simulink model "mdaqdemo_uart"  (R2014a)
settings: Solver=FixedStepDiscrete  SolverMode=SingleTasking  StartTime=0.0  StopTime=100  FixedStep=0.1  RelTol=1e-3
libraries: microdaq_lib x4, etargetslib x2, simulink x2
settings Model: SimulationMode=external  Creator=skibool  LastModifiedBy=skibool
settings OptimizationCC: OptimizeModelRefInitCode=on  LifeSpan=1
settings DebuggingCC: MergeDetectMultiDrivingBlocksExec=error  FrameProcessingCompatibilityMsg=error
settings HardwareCC: ProdBitPerLong=40  ProdLargestAtomicInteger=Integer  ProdIntDivRoundTo=Zero  ProdEndianess=LittleEndian  ProdHWDeviceType=Texas Instruments->C6000
settings RTWCC: SystemTargetFile=microdaq.tlc  TemplateMakefile=microdaq.tmf  PostCodeGenCommand=microdaq_postcodegen(buildInfo)  Description=MicroDAQ Real-Time Measurement System
settings CodeAppCC: IgnoreCustomStorageClasses=off
settings STFCustomTargetCC: ConcurrentExecutionCompliant=off  GeneratePreprocessorConditionals=Use local settings  CombineOutputUpdateFcns=on  ERTCustomFileBanners=on  SupportContinuousTime=off  SupportNonInlinedSFcns=off  MATLABClassNameForMDSCustomization=Simulink.SoftwareTarget.ERTCustomization  GRTInterface=off  SystemTargetFile=microdaq.tlc
settings ERTTargetCC: GenerateSampleERTMain=off  ExtMode=on  ExtModeStaticAlloc=on  ExtModeStaticAllocSize=1485760  ExtModeMexArgs=getpref('microdaq','TargetIP') 1 4344  InlinedParameterPlacement=Hierarchical  ERTCustomFileTemplate=microdaq_main.tlc

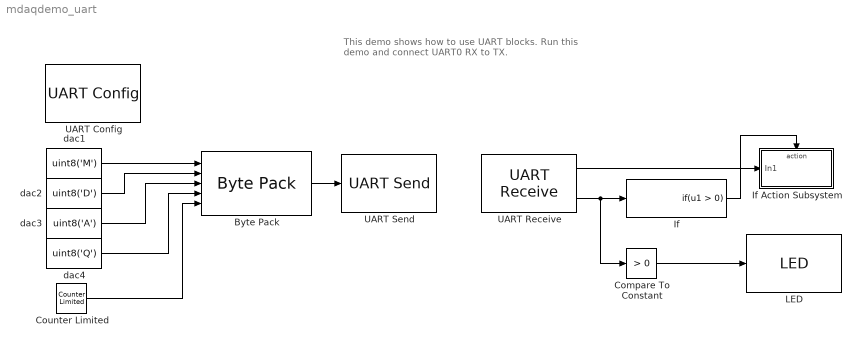
== system mdaqdemo_uart ==
  note: This demo shows how to use UART blocks.
      |
      | Run this demo and connect UART0 RX to TX.
  Byte Pack : etargetslib/Byte Pack  datatypes={'uint8','uint8','uint8','uint8', 'uint8'}  byteAlign=1
  Compare To Constant : simulink/Logic and Bit Operations/Compare To Constant  relop=>  const=0  OutDataTypeStr=uint8
  Counter Limited : simulink/Sources/Counter Limited  uplimit=100  tsamp=-1
  If : If  ShowElse=off
  If Action Subsystem : Subsystem  TreatAsAtomicUnit=on
  LED : microdaq_lib/Utilities/LED  SParameter1=D1
  UART Config : microdaq_lib/UART/UART Config  pModule=UART0  pBaudRate=9600  pDataBits=8  pParity=None  pStopBits=1  pFlowControl=None
  UART Receive : microdaq_lib/UART/UART Receive  pModule=UART0  pDataSize=5  pUseHeader=off  pHeaderStr=7161646d  pHeader=0  pBlocking=off  pTimeout=10  SampleTime=-1
  UART Send : microdaq_lib/UART/UART Send  pModule=UART0  pDataSize=5  SampleTime=-1
  dac1 : Constant  Value=uint8('M')  OutDataTypeStr=uint8
  dac2 : Constant  Value=uint8('D')  OutDataTypeStr=uint8
  dac3 : Constant  Value=uint8('A')  OutDataTypeStr=uint8
  dac4 : Constant  Value=uint8('Q')  OutDataTypeStr=uint8
  wires:
  If/1 -> If Action Subsystem/Action
  UART Receive/2 -> Compare To Constant/1, If/1
  UART Receive/1 -> If Action Subsystem/1(In1)
  Byte Pack/1 -> UART Send/1
  Compare To Constant/1 -> LED/1
  dac1/1 -> Byte Pack/1
  dac2/1 -> Byte Pack/2
  dac3/1 -> Byte Pack/3
  dac4/1 -> Byte Pack/4
  Counter Limited/1 -> Byte Pack/5

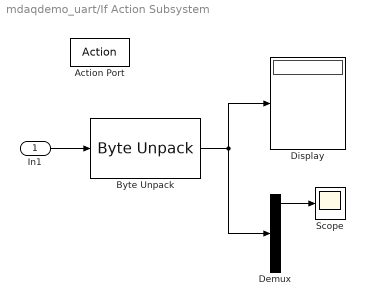
== system mdaqdemo_uart/If Action Subsystem ==
  In1 : Inport
  Action Port : ActionPort  ActionType=then
  Byte Unpack : etargetslib/Byte Unpack  dimensions={[5]}  datatypes={'uint8'}  byteAlign=1
  Demux : Demux  Outputs=5
  Display : Display
  Scope : Scope
      settings: TimeRange=auto  MaxDataPoints=5000  SaveToWorkspace=off  SaveName=ScopeData  YMin=-12.5  YMax=112.5  SampleTime=-1
  wires:
  In1/1 -> Byte Unpack/1
  Byte Unpack/1 -> Demux/1, Display/1
  Demux/1 -> Scope/1
